simulink model "neuron"  (Simulink 7.8)
settings: Solver=ode45  StartTime=0.0  StopTime=10.0  RelTol=1e-3
libraries: simulink x3
settings Model: Creator=Leo  LastModifiedBy=Leo

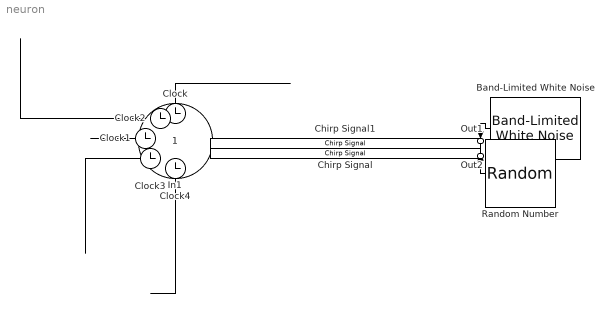
== system neuron ==
  In1 : Inport
  Band-Limited White Noise : simulink/Sources/Band-Limited White Noise  Cov=[0.1]  Ts=0.1  seed=[23341]
  Chirp Signal : simulink/Sources/Chirp Signal  f1=0.1  T=100  f2=1
  Chirp Signal1 : simulink/Sources/Chirp Signal  f1=0.1  T=100  f2=1
  Clock{,1..4} (5 alike) : Clock
  Random Number : RandomNumber  SampleTime=0.1
  Out1 : Outport
  Out2 : Outport  Port=2
  wires:
  Band-Limited White Noise/1 -> Out1/1
  Random Number/1 -> Out2/1
  Clock/1 -> ?
  Clock2/1 -> ?
  Clock1/1 -> ?
  Clock3/1 -> ?
  Clock4/1 -> ?
